simulink model "VDC_cont_4T_V3"  (R2019b)
settings: Solver=ode3  StartTime=0.0  StopTime=3  FixedStep=0.000050  RelTol=1e-3  EnableMultiTasking=on
settings Model: Creator=cary  LastModifiedBy=adshetgaonkar
settings DataIOCC: LimitDataPoints=on  SaveFormat=Array  SignalLoggingSaveFormat=ModelDataLogs  ReturnWorkspaceOutputs=off
settings OptimizationCC: ExpressionDepthLimit=2147483647  LifeSpan=1  EfficientTunableParamExpr=on
settings DebuggingCC: UnderspecifiedInitializationDetection=Classic  MergeDetectMultiDrivingBlocksExec=none  SolverPrmCheckMsg=warning  FcnCallInpInsideContextMsg=warning  StateNameClashWarn=warning  SFUnexpectedBacktrackingDiag=warning  SFNoUnconditionalDefaultTransitionDiag=warning  SFExecutionAtInitializationDiag=none  ArithmeticOperatorsInVariantConditions=warning
settings HardwareCC: ProdBitPerPointer=32  ProdBitPerSizeT=32  ProdBitPerPtrDiffT=32  ProdLargestAtomicFloat=None  ProdIntDivRoundTo=Undefined  ProdEndianess=Unspecified  ProdWordSize=32  ProdHWDeviceType=32-bit Generic
settings ModelReferenceCC: PropagateSignalLabelsOutOfModel=off
settings SFSimCC: SimUseLocalCustomCode=off  MATLABDynamicMemAlloc=off  CustomCodeUndefinedFunction=UseInterfaceOnly
settings RTWCC: SystemTargetFile=ert.tlc  TemplateMakefile=ert_default_tmf  RTWUseLocalCustomCode=off
settings CodeAppCC: IgnoreCustomStorageClasses=off  CustomSymbolStrType=$N$R$M  StateflowObjectComments=on  InternalIdentifier=Classic
settings ERTTargetCC: MultiwordLength=2048  GenerateSampleERTMain=on  IncludeMdlTerminateFcn=off  SupportComplex=off  SupportContinuousTime=on  ERTCustomFileTemplate=example_file_process.tlc  ConvertIfToSwitch=off  SuppressUnreachableDefaultCases=off
settings ConfigComp: CovMetricSettings=dw  CovHtmlReporting=on  CovSaveCumulativeToWorkspaceVar=on  CovSaveSingleToWorkspaceVar=on  CovExternalEMLEnable=off

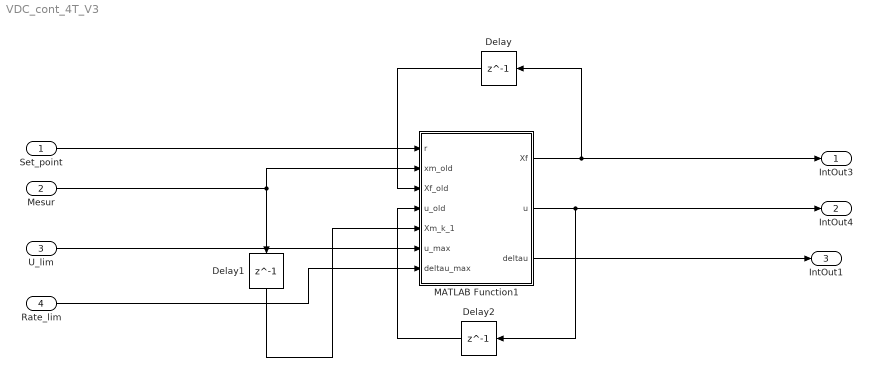
== system VDC_cont_4T_V3 ==
  Set_point : Inport
  Mesur : Inport  Port=2
  U_lim : Inport  Port=3
  Rate_lim : Inport  Port=4
  Delay : Delay  DelayLength=1  SampleTime=50e-6
  Delay1 : Delay  DelayLength=1  SampleTime=50e-6
  Delay2 : Delay  DelayLength=1  SampleTime=50e-6
  MATLAB Function1 : MATLAB Function  TreatAsAtomicUnit=on
  IntOut3 : Outport  SignalName=Xf
  IntOut4 : Outport  Port=2  SignalName=u
  IntOut1 : Outport  Port=3  SignalName=delta_u
  wires:
  Set_point/1 -> MATLAB Function1/1(r)
  MATLAB Function1/1(Xf) -> Delay/1, IntOut3/1
  MATLAB Function1/3(deltau) -> IntOut1/1
  Delay1/1 -> MATLAB Function1/5(Xm_k_1)
  Delay/1 -> MATLAB Function1/3(Xf_old)
  Mesur/1 -> MATLAB Function1/2(xm_old), Delay1/1
  MATLAB Function1/2(u) -> Delay2/1, IntOut4/1
  U_lim/1 -> MATLAB Function1/6(u_max)
  Rate_lim/1 -> MATLAB Function1/7(deltau_max)
  Delay2/1 -> MATLAB Function1/4(u_old)

== matlab function VDC_cont_4T_V3/MATLAB Function1 ==
  data: Xf output; r input; xm_old input; u output; Xf_old input; u_old input size=[1 1]; Xm_k_1 input; deltau output; u_max input; deltau_max input
function [Xf,u,deltau] = fcn(r,xm_old,Xf_old,u_old,Xm_k_1,u_max,deltau_max)

in = [];
%in = coder.load('Grid_forming.mat'); 
in = coder.load('4TDC_volatge.mat'); 
%% there is issue there which need to be fixed %%%
gamma=[(u_max - u_old);( u_max + u_old); deltau_max; deltau_max];
eta=QPhild(in.Omega,in.Psi*(in.Xf+Xf_old),in.M,gamma)
%%
%eta = -(in.Omega\in.Psi)*(in.Xf+Xf_old)  %%% original %%% 
deltau=in.Lzerot*eta; %%%% input signal 

%%
u=in.up+u_old+deltau;
%%%%
y = xm_old;
xm = xm_old;
y_delta_k = y-Xm_k_1;
Xf=[y_delta_k;y-r];
